simulink model "bank_model"  (R2019b)
settings: Solver=ode4  StartTime=0.0  StopTime=10.0  FixedStep=step_size  RelTol=1e-3
values from neighbouring files (symbols this model uses):
  A = lambda(i)    [Dyskretny.m]    (also in DyskretnyVsCiagly.m = expm(h*A_c); Kapitalizacja.m = 1.04)
  B = 0    [Dyskretny.m]    (also in DyskretnyVsCiagly.m = double(int(expm(t*A_c)*B_c,t,0,h)); Kapitalizacja.m)
  C = 1    [Dyskretny.m]    (also in DyskretnyVsCiagly.m = C_c; Kapitalizacja.m)
  D = 0    [Dyskretny.m]    (also in DyskretnyVsCiagly.m = D_c; Kapitalizacja.m)
  h = 1    [Dyskretny.m]    (also in DyskretnyVsCiagly.m; Kapitalizacja.m = cap_rate)
  Start = 10    [Dyskretny.m]    (also in DyskretnyVsCiagly.m = 5; Kapitalizacja.m = 10000)
  step_size = 0.01    [Kapitalizacja.m]
settings Model: Creator=bion  LastModifiedBy=resta
settings DataIOCC: ReturnWorkspaceOutputs=off
settings DebuggingCC: ArithmeticOperatorsInVariantConditions=warning
settings SFSimCC: CustomCodeUndefinedFunction=UseInterfaceOnly

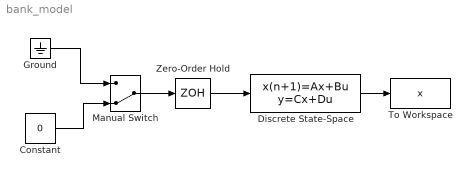
== system bank_model ==
  Constant : Constant  Value=0  SampleTime=h
  Discrete State-Space : DiscreteStateSpace  A=A  B=B  C=C  D=D  InitialCondition=Start  SampleTime=h
  Ground : Ground
  Manual Switch : ManualSwitch  CurrentSetting=0
  To Workspace : ToWorkspace  VariableName=x  SampleTime=step_size
  Zero-Order Hold : ZeroOrderHold  SampleTime=h
  wires:
  Constant/1 -> Manual Switch/2
  Zero-Order Hold/1 -> Discrete State-Space/1
  Discrete State-Space/1 -> To Workspace/1
  Manual Switch/1 -> Zero-Order Hold/1
  Ground/1 -> Manual Switch/1
